simulink model "preliminaryModel_noBS13"  (R2015b)
settings: Solver=FixedStepAuto  StartTime=cmd_time(1215)  StopTime=cmd_time(1215)+10  FixedStep=1E-2  MaxStep=0.08  RelTol=1e-3
values from neighbouring files (symbols this model uses):
  act_0 = 0.3    [runfirst13.m]
  b = 1.365    [runfirst13.m]
  cbar = 0.5    [runfirst13.m]
  CD_alpha = 0.173    [runfirst13.m]
  CD_beta = 0    [runfirst13.m]
  CD_ca = 0    [runfirst13.m]
  CD_el = 0    [runfirst13.m]
  CG = [Xcg Ycg Zcg]    [runfirst13.m]
  CL_alpha = 3.137    [runfirst13.m]
  Cl_alpha = 0    [runfirst13.m]
  Cl_beta = 0.046    [runfirst13.m]
  CL_beta = 0    [runfirst13.m]
  CL_ca = 0.000    (= 0)    [runfirst13.m]
  Cl_ca = 0.000    (= 0)    [runfirst13.m]
  CL_el = 0.000    (= 0)    [runfirst13.m]
  Cl_el = 0.111    [runfirst13.m]
  Cm_alpha = -0.083    [runfirst13.m]
  Cm_beta = 0    [runfirst13.m]
  Cm_ca = -0.456    [runfirst13.m]
  Cm_el = 0.000    (= 0)    [runfirst13.m]
  Cn_alpha = 0    [runfirst13.m]
  Cn_beta = 0    [runfirst13.m]
  Cn_ca = 0.000    (= 0)    [runfirst13.m]
  Cn_el = 0.037    [runfirst13.m]
  CP = [xa_ref 0 0]    [runfirst13.m]
  CY_alpha = 0    [runfirst13.m]
  CY_beta = -0.351    [runfirst13.m]
  CY_ca = 0.000    (= 0)    [runfirst13.m]
  CY_el = 0.049    [runfirst13.m]
  deg_2_rad = 1/rad_2_deg    (= 0.0174532925199)    [runfirst13.m]
  eul_0 = [phi_0 theta_0 psi_0]    [runfirst13.m]
  f = 1/196.877360    (= 0.00507930419221)    [runfirst13.m]
  F_0 = [100 0 0]    [runfirst13.m]
  g = 9.82    [runfirst13.m]
  h_ref = 0    [runfirst13.m]
  heading_0 = 0    [runfirst13.m]
  Iyy = 0.01    [runfirst13.m]
  LL0 = [1 0]    [runfirst13.m]
  m_dot = 0.2    [runfirst13.m]
  mass = W_oew    (= 14.95)    [runfirst13.m]
  mass_e = 0    [runfirst13.m]
  mass_f = mass+W_if    (= 17.85)    [runfirst13.m]
  maxdef_act = 2.0    (= 2)    [runfirst13.m]
  maxrate_act = inf    [runfirst13.m]
  mindef_act = -2.0    (= -2)    [runfirst13.m]
  P_g = 100000    [runfirst13.m]
  pos3_0 = [Xe_0 Ze_0]    [runfirst13.m]
  pos_0 = [Xe_0 Ye_0 Ze_0]    [runfirst13.m]
  q_0 = 0.5    [runfirst13.m]
  R = 287    [runfirst13.m]
  rad_2_deg = 180/pi    (= 57.2957795131)    [runfirst13.m]
  rho_ref = 1.225    [runfirst13.m]
  rot_0 = [p_0 q_0 r_0]    [runfirst13.m]
  S_ref = 0.747    [runfirst13.m]
  T_g = 293    [runfirst13.m]
  theta_0 = 0.02    [runfirst13.m]
  U_0 = 10    [runfirst13.m]
  Vb_0 = [U_0 v_0 w_0]    [runfirst13.m]
  Vw_0 = [uw_0 vw_0 ww_0]    [runfirst13.m]
  w_0 = 0    [runfirst13.m]
  wn_act = 1.7    [runfirst13.m]
  z_act = 0.57    [runfirst13.m]
undefined symbols (not defined in the file or in its folder): Newton, Raphson, U0, w0
libraries: simulink x6
(part 1 of 2)
settings Model: Creator=Victor  LastModifiedBy=victorohman
settings OptimizationCC: BlockReduction=off  UseDivisionForNetSlopeComputation=on  EfficientFloat2IntCast=on
settings DebuggingCC: SignalInfNanChecking=error  SignalRangeChecking=error  ReadBeforeWriteMsg=EnableAllAsError  WriteAfterWriteMsg=EnableAllAsError  WriteAfterReadMsg=EnableAllAsError  AlgebraicLoopMsg=error  ArtificialAlgebraicLoopMsg=error  BlockPriorityViolationMsg=error  SolverPrmCheckMsg=error  InheritedTsInSrcMsg=error  SigSpecEnsureSampleTimeMsg=error  CheckMatrixSingularityMsg=error  IntegerOverflowMsg=error  ParameterUnderflowMsg=error  ParameterPrecisionLossMsg=error  ParameterTunabilityLossMsg=error  UnderSpecifiedDataTypeMsg=error  UnnecessaryDatatypeConvMsg=warning  SignalLabelMismatchMsg=error  UnconnectedInputMsg=error  UnconnectedOutputMsg=error  UnconnectedLineMsg=error  UniqueDataStoreMsg=error  BusObjectLabelMismatch=error  RootOutportRequireBusObject=error  AssertControl=DisableAll  UnknownTsInhSupMsg=error  StateNameClashWarn=warning  StrictBusMsg=ErrorOnBusTreatedAsVector
settings GRTTargetCC: UtilityFuncGeneration=Shared location

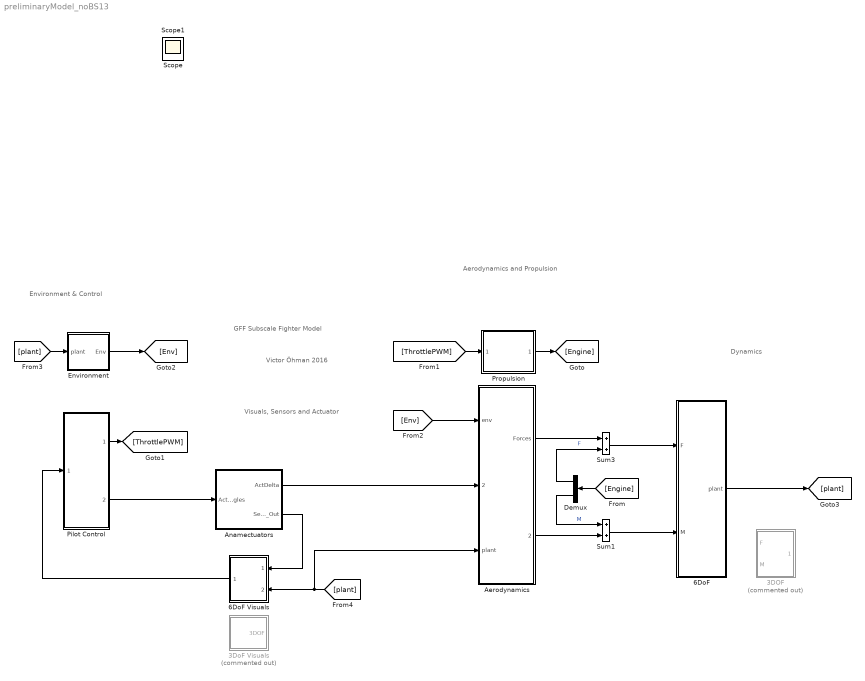
== system preliminaryModel_noBS13 ==
  note: Victor Öhman
      | 2016
  note: GFF
      | Subscale Fighter Model
  note: Environment & Control
  note: Visuals, Sensors
      | and Actuator
  note: Aerodynamics
      | and Propulsion
  note: Dynamics
  3DOF : Subsystem  Commented=on  VariantControl=Variant1
  3DoF Visuals : Subsystem  Commented=on
  6DoF : Subsystem
  6DoF Visuals : Subsystem
  Aerodynamics : Subsystem
  Anamectuators : Subsystem
  Demux : Demux  Outputs=2
  Environment : Subsystem
  Pilot Control : Subsystem
  Propulsion : Subsystem
  Sum1 : Sum  SaturateOnIntegerOverflow=on  InputSameDT=on  OutDataTypeStr=Inherit: Same as first input
  Sum3 : Sum  SaturateOnIntegerOverflow=on  InputSameDT=on  OutDataTypeStr=Inherit: Same as first input
  Scope : Scope
  Scope1 : Scope
  wires:
  Pilot Control/2(ActPos) -> Anamectuators/1(ActCmdAngles)
  Anamectuators/2(Sensor_Out) -> 6DoF Visuals/1(Sensors)
  Propulsion/1(Engine) -> [Engine]
  Aerodynamics/2(Moments) -> Sum1/2
  Aerodynamics/1(Forces) -> Sum3/1
  Demux/1 -> Sum3/2  "F"
  Demux/2 -> Sum1/1  "M"
  Anamectuators/1(ActDelta) -> Aerodynamics/2(ActDelta)
  Sum1/1 -> 6DoF/2(M)
  Sum3/1 -> 6DoF/1(F)
  [Engine] -> Demux/1
  Pilot Control/1(Throttle,PWM) -> [ThrottlePWM]
  [ThrottlePWM] -> Propulsion/1(Throttle)
  Environment/1(Env) -> [Env]
  [Env] -> Aerodynamics/1(env)
  6DoF/1(plant) -> [plant]
  [plant] -> Environment/1(plant)
  [plant] -> Aerodynamics/3(plant), 6DoF Visuals/2(6DOF)
  6DoF Visuals/1(Autopilot) -> Pilot Control/1(Autopilot)

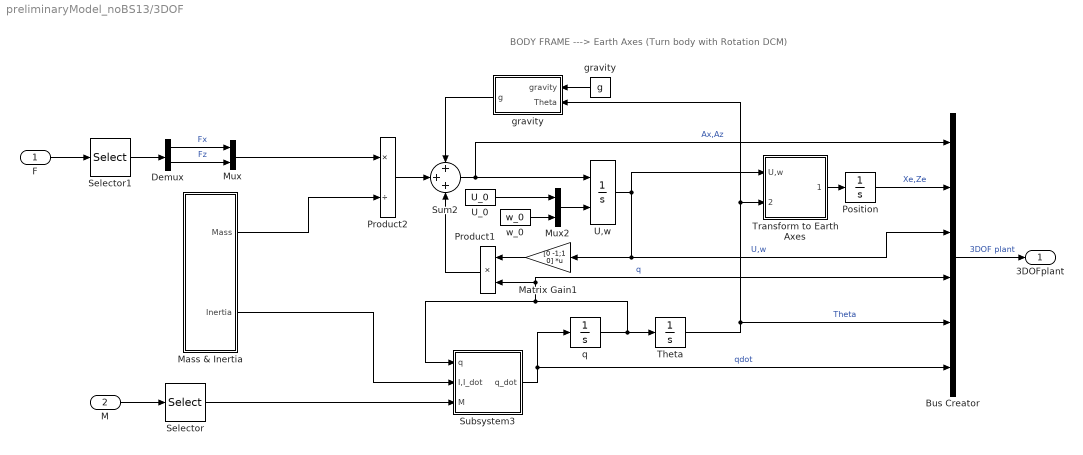
== system preliminaryModel_noBS13/3DOF ==
  note: BODY FRAME ---> Earth Axes (Turn body with Rotation DCM)
  F : Inport
  M : Inport  Port=2
  Bus Creator : BusCreator  Inputs=6
  Demux : Demux  Outputs=2
  Mass & Inertia : Subsystem
  Matrix Gain1 : Gain  Gain=[0 -1;1 0]  Multiplication=Matrix(K*u)  SaturateOnIntegerOverflow=on  OutDataTypeStr=Inherit: Same as input  ParamDataTypeStr=Inherit: Same as input
  Mux : Mux  Inputs=2
  Mux2 : Mux  Inputs=2
  Position : Integrator  InitialCondition=pos3_0
  Product1 : Product  SaturateOnIntegerOverflow=on  InputSameDT=on  OutDataTypeStr=Inherit: Same as first input
  Product2 : Product  Inputs=*/  SaturateOnIntegerOverflow=on  OutDataTypeStr=Inherit: Same as first input
  Selector : Selector  IndexMode=Zero-based  InputPortWidth=3  IndexOptions=Index vector (dialog)  Indices=1  OutputSizes=1
  Selector1 : Selector  InputPortWidth=3  IndexOptions=Index vector (dialog)  Indices=[1 3]  OutputSizes=1
  Subsystem3 : Subsystem
  Sum2 : Sum  Inputs=+++  SaturateOnIntegerOverflow=on
  Theta : Integrator  InitialCondition=theta_0
  Transform to Earth Axes : Subsystem
  U,w : Integrator  InitialConditionSource=external  InitialCondition=convvel([U0 w0],'m/s','m/s')
  U_0 : Constant  Value=U_0
  gravity : Constant  Value=g  OutDataTypeStr=Inherit: Inherit via back propagation
  "gravity " : Subsystem
  q : Integrator  InitialCondition=q_0
  w_0 : Constant  Value=w_0
  3DOFplant : Outport
  wires:
  Bus Creator/1 -> 3DOFplant/1  "3DOF plant"
  Mux2/1 -> U,w/2
  U_0/1 -> Mux2/1
  w_0/1 -> Mux2/2
  Selector/1 -> Subsystem3/3(M)
  U,w/1 -> Matrix Gain1/1, Bus Creator/3, Transform to Earth Axes/1(U,w)  "U,w"
  gravity/1 -> "gravity "/1(gravity)
  Mass & Inertia/2(Inertia) -> Subsystem3/2(I,I_dot)
  Mass & Inertia/1(Mass) -> Product2/2
  Sum2/1 -> U,w/1, Bus Creator/1  "Ax,Az"
  q/1 -> Subsystem3/1(q), Product1/2, Bus Creator/4, Theta/1  "q"
  Subsystem3/1(q_dot) -> q/1, Bus Creator/6  "qdot"
  Theta/1 -> "gravity "/2(Theta), Transform to Earth Axes/2(Theta), Bus Creator/5  "Theta"
  Position/1 -> Bus Creator/2  "Xe,Ze"
  Matrix Gain1/1 -> Product1/1
  Transform to Earth Axes/1(Ue,we) -> Position/1
  Product1/1 -> Sum2/3
  Product2/1 -> Sum2/2
  "gravity "/1(g) -> Sum2/1
  Mux/1 -> Product2/1
  Selector1/1 -> Demux/1
  Demux/2 -> Mux/2  "Fz"
  Demux/1 -> Mux/1  "Fx"
  F/1 -> Selector1/1
  M/1 -> Selector/1

== system preliminaryModel_noBS13/3DoF Visuals ==
  3DOF : Inport
  Bus Selector1 : BusSelector  OutputSignals=Xe;Ze
  Mux1 : Mux  Inputs=1
  To File : ToFile  Filename=output_3dof.mat  SaveFormat=Timeseries
  lat : Scope
  wires:
  3DOF/1 -> Bus Selector1/1
  Mux1/1 -> To File/1
  Bus Selector1/1 -> lat/1, Mux1/1  "<Xe;Ze>"

== system preliminaryModel_noBS13/6DoF ==
  F : Inport
  M : Inport  Port=2
  "  " : Subsystem
  "        " : Subsystem
  "               " : Subsystem
  " 1" : Subsystem
  6DOF : Subsystem
  Bus Creator : BusCreator  Inputs=9
  plant : Outport
  wires:
  F/1 -> 6DOF/1(F)
  "  "/1(body angles) -> Bus Creator/3
  " 1"/1(NED pos) -> Bus Creator/9  "NED pos"
  Bus Creator/1 -> plant/1
  6DOF/8(Xe) -> Bus Creator/8, " 1"/1(Xe)  "Xe"
  "        "/1(omega) -> Bus Creator/5  "w"
  6DOF/1(Ve) -> Bus Creator/1  "Ve"
  6DOF/7(Ab) -> Bus Creator/7  "Ab"
  "               "/1(omegadot) -> Bus Creator/6  "wdot"
  6DOF/2(Vb) -> Bus Creator/2  "Vb"
  6DOF/3(Euler) -> "  "/1(phi,theta,psi)
  6DOF/6(pdot,qdot,rdot) -> "               "/1(pdot,qdot,rdot)
  6DOF/4(DCM) -> Bus Creator/4  "DCM"
  6DOF/5(p,q,r) -> "        "/1(p,q,r)
  M/1 -> 6DOF/2(M)

== system preliminaryModel_noBS13/6DoF Visuals ==
  note: Block för att kolla, skicka vidare
  Sensors : Inport
  6DOF : Inport  Port=2
  Bus Selector2 : BusSelector  OutputSignals=NED pos.lat,NED pos.long,NED pos.alt,body angles.phi,body angles.theta,body angles.psi
  Mux1 : Mux  Inputs=3
  Mux2 : Mux  Inputs=3
  Scope : Scope  NumInputPorts=3
  To File : ToFile  Filename=out_pos.mat  MatrixName=out_pos  SaveFormat=Timeseries
  To File1 : ToFile  Filename=out_eul.mat  MatrixName=out_eul  SaveFormat=Timeseries
  alt : Scope
  lat : Scope
  long : Scope
  Autopilot : Outport
  wires:
  Bus Selector2/4 -> Mux2/1, Scope/1  "<phi>"
  Bus Selector2/6 -> Mux2/3, Scope/3  "<psi>"
  6DOF/1 -> Bus Selector2/1
  Bus Selector2/5 -> Mux2/2, Scope/2  "<theta>"
  Bus Selector2/2 -> Mux1/2, long/1  "<long>"
  Bus Selector2/1 -> Mux1/1, lat/1  "<lat>"
  Bus Selector2/3 -> Mux1/3, alt/1  "<alt>"
  Mux1/1 -> To File/1
  Mux2/1 -> To File1/1
  Sensors/1 -> Autopilot/1

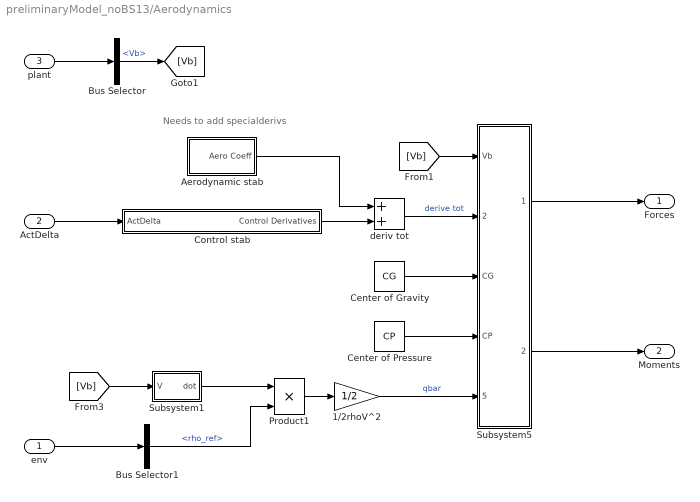
== system preliminaryModel_noBS13/Aerodynamics ==
  note: Needs to add specialderivs
  env : Inport
  ActDelta : Inport  Port=2
  plant : Inport  Port=3
  1/2rhoV^2 : Gain  Gain=1/2  SaturateOnIntegerOverflow=on  OutDataTypeStr=Inherit: Same as input  ParamDataTypeStr=Inherit: Same as input
  Aerodynamic stab : Subsystem
  Bus Selector : BusSelector  OutputSignals=Vb
  Bus Selector1 : BusSelector  OutputSignals=rho_ref
  Center of Gravity : Constant  Value=CG
  Center of Pressure : Constant  Value=CP
  Control stab : Subsystem
  Product1 : Product  SaturateOnIntegerOverflow=on  InputSameDT=on  OutDataTypeStr=Inherit: Same as first input
  Subsystem1 : Subsystem
  Subsystem5 : Subsystem
  deriv tot : Sum  SaturateOnIntegerOverflow=on  InputSameDT=on  OutDataTypeStr=Inherit: Same as first input
  Forces : Outport
  Moments : Outport  Port=2
  wires:
  plant/1 -> Bus Selector/1
  ActDelta/1 -> Control stab/1(ActDelta)
  env/1 -> Bus Selector1/1
  Bus Selector/1 -> [Vb]  "<Vb>"
  Aerodynamic stab/1(Aero Coeff) -> deriv tot/1
  Control stab/1(Control Derivatives) -> deriv tot/2
  Bus Selector1/1 -> Product1/2  "<rho_ref>"
  Product1/1 -> 1/2rhoV^2/1
  Subsystem1/1(dot) -> Product1/1
  [Vb] -> Subsystem1/1(V)
  Center of Gravity/1 -> Subsystem5/3(CG)
  deriv tot/1 -> Subsystem5/2(coef)  "derive tot"
  Center of Pressure/1 -> Subsystem5/4(CP)
  1/2rhoV^2/1 -> Subsystem5/5(qbar)  "qbar"
  Subsystem5/2(Moments) -> Moments/1
  Subsystem5/1(Forces) -> Forces/1
  [Vb] -> Subsystem5/1(Vb)

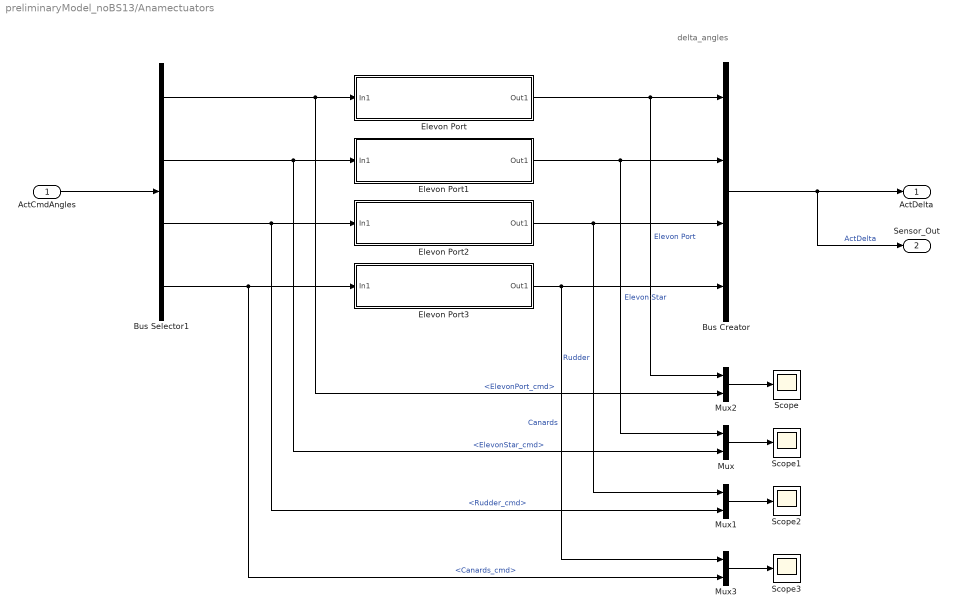
== system preliminaryModel_noBS13/Anamectuators ==
  note: delta_angles
  ActCmdAngles : Inport
  Bus Creator : BusCreator  Inputs=4
  Bus Selector1 : BusSelector  OutputSignals=ElevonPort_cmd,ElevonStar_cmd,Rudder_cmd,Canards_cmd
  Elevon Port : Subsystem
  Elevon Port1 : Subsystem
  Elevon Port2 : Subsystem
  Elevon Port3 : Subsystem
  Mux{,1..3} (4 alike) : Mux  Inputs=2
  Scope{,1..3} (4 alike) : Scope
  ActDelta : Outport
  Sensor_Out : Outport  Port=2
  wires:
  ActCmdAngles/1 -> Bus Selector1/1
  Bus Selector1/1 -> Elevon Port/1(In1), Mux2/2  "<ElevonPort_cmd>"
  Bus Selector1/2 -> Elevon Port1/1(In1), Mux/2  "<ElevonStar_cmd>"
  Bus Selector1/3 -> Elevon Port2/1(In1), Mux1/2  "<Rudder_cmd>"
  Bus Creator/1 -> Sensor_Out/1, ActDelta/1  "ActDelta"
  Mux/1 -> Scope1/1
  Mux1/1 -> Scope2/1
  Mux2/1 -> Scope/1
  Mux3/1 -> Scope3/1
  Bus Selector1/4 -> Elevon Port3/1(In1), Mux3/2  "<Canards_cmd>"
  Elevon Port/1(Out1) -> Bus Creator/1, Mux2/1  "Elevon Port"
  Elevon Port1/1(Out1) -> Bus Creator/2, Mux/1  "Elevon Star"
  Elevon Port2/1(Out1) -> Bus Creator/3, Mux1/1  "Rudder"
  Elevon Port3/1(Out1) -> Bus Creator/4, Mux3/1  "Canards"

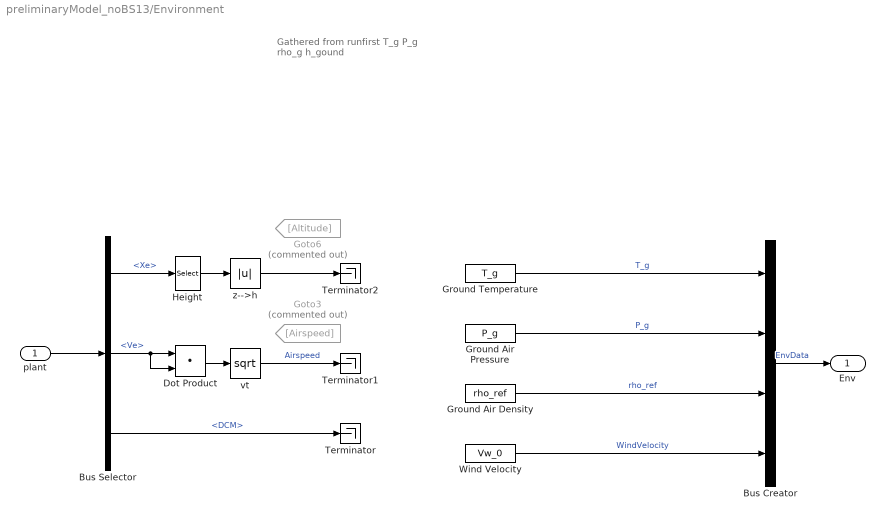
== system preliminaryModel_noBS13/Environment ==
  note: Gathered from runfirst
      | T_g
      | P_g
      | rho_g
      | h_gound
  plant : Inport
  Bus Creator : BusCreator  Inputs='T_g','P_g','rho_ref','WindVelocity'
  Bus Selector : BusSelector  OutputSignals=Xe,Ve,DCM
  Dot Product : DotProduct  OutDataTypeStr=Inherit: Inherit via internal rule
  Goto3 : Goto  Commented=on  GotoTag=Airspeed
  Goto6 : Goto  Commented=on  GotoTag=Altitude
  Ground Air Density : Constant  Value=rho_ref
  Ground Air Pressure : Constant  Value=P_g
  Ground Temperature : Constant  Value=T_g
  Height : Selector  InputPortWidth=3  IndexOptions=Index vector (dialog)  Indices=[3]  OutputSizes=1
  Terminator : Terminator
  Terminator1 : Terminator
  Terminator2 : Terminator
  Wind Velocity : Constant  Value=Vw_0
  vt : Math  Operator=sqrt  SaturateOnIntegerOverflow=on
  z-->h : Abs  SaturateOnIntegerOverflow=on
  Env : Outport  InitialOutput=0
  wires:
  Bus Creator/1 -> Env/1  "EnvData"
  Ground Temperature/1 -> Bus Creator/1  "T_g"
  Ground Air Pressure/1 -> Bus Creator/2  "P_g"
  Bus Selector/3 -> Terminator/1  "<DCM>"
  Height/1 -> z-->h/1
  Ground Air Density/1 -> Bus Creator/3  "rho_ref"
  z-->h/1 -> Terminator2/1
  Bus Selector/1 -> Height/1  "<Xe>"
  plant/1 -> Bus Selector/1
  vt/1 -> Terminator1/1  "Airspeed"
  Dot Product/1 -> vt/1
  Wind Velocity/1 -> Bus Creator/4  "WindVelocity"
  Bus Selector/2 -> Dot Product/2, Dot Product/1  "<Ve>"

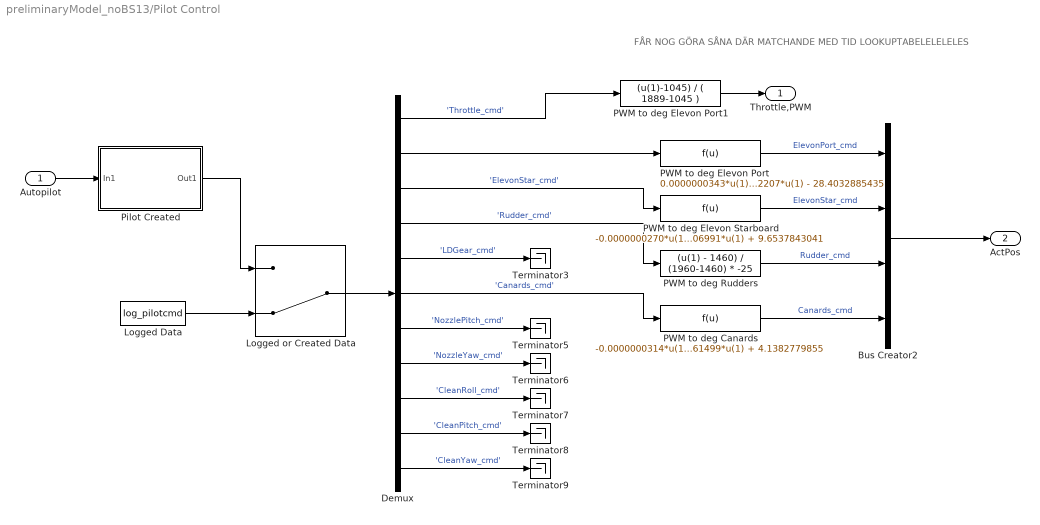
== system preliminaryModel_noBS13/Pilot Control ==
  note: FÅR NOG GÖRA SÅNA DÄR MATCHANDE MED TID LOOKUPTABELELELELES
  Autopilot : Inport
  Bus Creator2 : BusCreator  Inputs=4
  Demux : Demux  Outputs=11
  Logged Data : FromWorkspace  VariableName=log_pilotcmd  SampleTime=0
  Logged or Created Data : ManualSwitch  CurrentSetting=0
  PWM to deg Canards : Fcn  Expr=-0.0000000314*u(1)^3 + 0.0001339606*u(1)^2 - 0.1313561499*u(1) + 4.1382779855
  PWM to deg Elevon Port : Fcn  Expr=0.0000000343*u(1)^3 - 0.0001530183*u(1)^2 + 0.1711412207*u(1) - 28.4032885435
  PWM to deg Elevon Port1 : Fcn  Expr=(u(1)-1045) / ( 1889-1045 )
  PWM to deg Elevon Starboard : Fcn  Expr=-0.0000000270*u(1)^3 + 0.0001190841*u(1)^2 - 0.1226606991*u(1) + 9.6537843041
  PWM to deg Rudders : Fcn  Expr=(u(1) - 1460) / (1960-1460) * -25
  Pilot Created : Subsystem
  Terminator{3,5..9} (6 alike) : Terminator
  Throttle,PWM : Outport
  ActPos : Outport  Port=2
  wires:
  Bus Creator2/1 -> ActPos/1
  PWM to deg Canards/1 -> Bus Creator2/4  "Canards_cmd"
  PWM to deg Elevon Port/1 -> Bus Creator2/1  "ElevonPort_cmd"
  PWM to deg Elevon Starboard/1 -> Bus Creator2/2  "ElevonStar_cmd"
  PWM to deg Rudders/1 -> Bus Creator2/3  "Rudder_cmd"
  Logged Data/1 -> Logged or Created Data/2
  Demux/1 -> PWM to deg Elevon Port1/1  "'Throttle_cmd'"
  Demux/2 -> PWM to deg Elevon Port/1
  Demux/3 -> PWM to deg Elevon Starboard/1  "'ElevonStar_cmd'"
  Demux/4 -> PWM to deg Rudders/1  "'Rudder_cmd'"
  Demux/5 -> Terminator3/1  "'LDGear_cmd'"
  Demux/6 -> PWM to deg Canards/1  "'Canards_cmd'"
  Demux/7 -> Terminator5/1  "'NozzlePitch_cmd'"
  Demux/8 -> Terminator6/1  "'NozzleYaw_cmd'"
  Demux/9 -> Terminator7/1  "'CleanRoll_cmd'"
  Demux/10 -> Terminator8/1  "'CleanPitch_cmd'"
  Demux/11 -> Terminator9/1  "'CleanYaw_cmd'"
  Logged or Created Data/1 -> Demux/1
  Pilot Created/1(Out1) -> Logged or Created Data/1
  Autopilot/1 -> Pilot Created/1(In1)
  PWM to deg Elevon Port1/1 -> Throttle,PWM/1

== system preliminaryModel_noBS13/Propulsion ==
  Throttle : Inport
  Engine Input : Subsystem
      settings: RTWSystemCode=Inline
  Mux4 : Mux  Inputs=2
  Engine : Outport
  wires:
  Throttle/1 -> Engine Input/1(throttle)
  Engine Input/2(M) -> Mux4/2
  Engine Input/1(F) -> Mux4/1
  Mux4/1 -> Engine/1

== system preliminaryModel_noBS13/3DOF/Mass & Inertia ==
  Constant : Constant  Value=Iyy  OutDataTypeStr=double
  Constant2 : Constant  Value=0  OutDataTypeStr=double
  Mux1 : Mux  Inputs=2
  mass1 : Integrator  InitialCondition=mass  LimitOutput=on  UpperSaturationLimit=mass_f  LowerSaturationLimit=mass_e
  massflow : Constant  Value=m_dot  OutDataTypeStr=Inherit: Inherit via back propagation
  Mass : Outport
  Inertia : Outport  Port=2
  wires:
  Constant2/1 -> Mux1/2
  Constant/1 -> Mux1/1
  massflow/1 -> mass1/1
  Mux1/1 -> Inertia/1
  mass1/1 -> Mass/1

== system preliminaryModel_noBS13/3DOF/Subsystem3 ==
  q : Inport
  I,I_dot : Inport  Port=2
  M : Inport  Port=3
  Demux : Demux  Outputs=2
  Product3 : Product  Inputs=*/  SaturateOnIntegerOverflow=on  InputSameDT=on  OutDataTypeStr=Inherit: Same as first input
  Product4 : Product  SaturateOnIntegerOverflow=on  InputSameDT=on  OutDataTypeStr=Inherit: Same as first input
  Sum2 : Sum  Inputs=|+-  SaturateOnIntegerOverflow=on
  q_dot : Outport
  wires:
  Demux/2 -> Product4/1
  I,I_dot/1 -> Demux/1
  Product4/1 -> Sum2/2
  q/1 -> Product4/2
  M/1 -> Sum2/1
  Product3/1 -> q_dot/1
  Demux/1 -> Product3/2
  Sum2/1 -> Product3/1

== system preliminaryModel_noBS13/3DOF/Transform to Earth Axes ==
  note: Rotation order ZYX
  U,w : Inport
  Theta : Inport  Port=2
  Constant : Constant  Value=0
  Mux3 : Mux  Inputs=3
  Mux4 : Mux  Inputs=3
  Product : Product  Multiplication=Matrix(*)  SaturateOnIntegerOverflow=on  OutDataTypeStr=Inherit: Same as first input
  Rotation Angles to Direction Cosine Matrix : Subsystem
  Selector : Selector  IndexMode=Zero-based  InputPortWidth=2  IndexOptions=Index vector (dialog)  Indices=0  OutputSizes=1
  Selector1 : Selector  InputPortWidth=3  IndexOptions=Index vector (dialog)  Indices=[1 3]  OutputSizes=1
  Selector2 : Selector  InputPortWidth=2  IndexOptions=Index vector (dialog)  Indices=2  OutputSizes=1
  Transpose : Math  Operator=transpose  SaturateOnIntegerOverflow=on
  Ue,we : Outport
  wires:
  Selector/1 -> Mux4/1
  Mux4/1 -> Product/2
  Transpose/1 -> Product/1  "DCMeb"
  Product/1 -> Selector1/1
  Theta/1 -> Mux3/2
  Rotation Angles to Direction Cosine Matrix/1(DCMbe) -> Transpose/1
  Mux3/1 -> Rotation Angles to Direction Cosine Matrix/1("[R1,R2,R3]")
  Selector1/1 -> Ue,we/1
  U,w/1 -> Selector/1, Selector2/1
  Selector2/1 -> Mux4/3
  Constant/1 -> Mux3/1, Mux3/3, Mux4/2

== system preliminaryModel_noBS13/3DOF/gravity  ==
  gravity : Inport
  Theta : Inport  Port=2
  Mux : Mux  Inputs=2
  Product : Product  SaturateOnIntegerOverflow=on  InputSameDT=on  OutDataTypeStr=Inherit: Same as first input
  Unary Minus : UnaryMinus
  sincos : Trigonometry  Operator=sincos
  g : Outport
  wires:
  sincos/1 -> Unary Minus/1
  sincos/2 -> Mux/2
  gravity/1 -> Product/2
  Theta/1 -> sincos/1
  Mux/1 -> Product/1
  Product/1 -> g/1
  Unary Minus/1 -> Mux/1

== system preliminaryModel_noBS13/6DoF/   ==
  phi,theta,psi : Inport
  Bus Creator1 : BusCreator  Inputs=3
  Demux3 : Demux  Outputs=3
  body angles : Outport
  wires:
  Demux3/2 -> Bus Creator1/2  "theta"
  Bus Creator1/1 -> body angles/1  "body angles"
  Demux3/3 -> Bus Creator1/3  "psi"
  phi,theta,psi/1 -> Demux3/1
  Demux3/1 -> Bus Creator1/1  "phi"

== system preliminaryModel_noBS13/6DoF/         ==
  p,q,r : Inport
  Bus Creator2 : BusCreator  Inputs=3
  Demux1 : Demux  Outputs=3
  omega : Outport
  wires:
  p,q,r/1 -> Demux1/1
  Bus Creator2/1 -> omega/1
  Demux1/3 -> Bus Creator2/3  "r"
  Demux1/1 -> Bus Creator2/1  "p"
  Demux1/2 -> Bus Creator2/2  "q"

== system preliminaryModel_noBS13/6DoF/                ==
  pdot,qdot,rdot : Inport
  Bus Creator2 : BusCreator  Inputs=3
  Demux1 : Demux  Outputs=3
  omegadot : Outport
  wires:
  pdot,qdot,rdot/1 -> Demux1/1
  Bus Creator2/1 -> omegadot/1
  Demux1/3 -> Bus Creator2/3  "rdot"
  Demux1/1 -> Bus Creator2/1  "pdot"
  Demux1/2 -> Bus Creator2/2  "qdot"

== system preliminaryModel_noBS13/6DoF/ 1 ==
  Xe : Inport
  Bus Creator : BusCreator  Inputs=3
  Constant : Constant  Value=h_ref
  Demux2 : Demux  Outputs=2
  Flat Earth to LLA : Subsystem
  NED pos : Outport
  wires:
  Xe/1 -> Flat Earth to LLA/1(Xe)
  Bus Creator/1 -> NED pos/1
  Constant/1 -> Flat Earth to LLA/2(ground height)
  Flat Earth to LLA/2(h) -> Bus Creator/3  "alt"
  Flat Earth to LLA/1(mu l) -> Demux2/1
  Demux2/1 -> Bus Creator/1  "lat"
  Demux2/2 -> Bus Creator/2  "long"

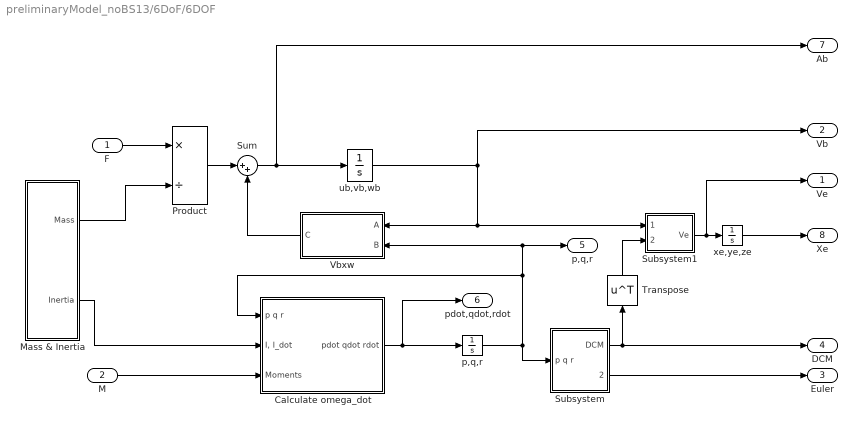
== system preliminaryModel_noBS13/6DoF/6DOF ==
  F : Inport
  M : Inport  Port=2
  Calculate omega_dot : Subsystem
  Mass & Inertia : Subsystem
  Product : Product  Inputs=*/  SaturateOnIntegerOverflow=on  OutDataTypeStr=Inherit: Same as first input
  Subsystem : Subsystem
  Subsystem1 : Subsystem
  Sum : Sum  Inputs=|++  SaturateOnIntegerOverflow=on
  Transpose : Math  Operator=transpose  SaturateOnIntegerOverflow=on
  Vbxw : Subsystem
  "p,q,r " : Integrator  InitialCondition=rot_0
  ub,vb,wb : Integrator  InitialCondition=Vb_0
  xe,ye,ze : Integrator  InitialCondition=pos_0
  Ve : Outport
  Vb : Outport  Port=2
  Euler : Outport  Port=3
  DCM : Outport  Port=4
  p,q,r : Outport  Port=5
  pdot,qdot,rdot : Outport  Port=6
  Ab : Outport  Port=7
  Xe : Outport  Port=8
  wires:
  Subsystem1/1(Ve) -> Ve/1, xe,ye,ze/1
  Sum/1 -> Ab/1, ub,vb,wb/1
  ub,vb,wb/1 -> Vb/1, Subsystem1/1(x y z), Vbxw/1(A)
  Calculate omega_dot/1(pdot qdot rdot) -> pdot,qdot,rdot/1, "p,q,r "/1
  Transpose/1 -> Subsystem1/2(transform coefficients)
  Subsystem/1(DCM) -> Transpose/1, DCM/1
  Product/1 -> Sum/1
  M/1 -> Calculate omega_dot/3(Moments)
  "p,q,r "/1 -> Subsystem/1("p q r "), p,q,r/1, Vbxw/2(B), Calculate omega_dot/1(p q r)
  xe,ye,ze/1 -> Xe/1
  Vbxw/1(C) -> Sum/2
  Subsystem/2(Euler) -> Euler/1
  Mass & Inertia/1(Mass) -> Product/2
  F/1 -> Product/1
  Mass & Inertia/2(Inertia) -> Calculate omega_dot/2("I, I_dot")

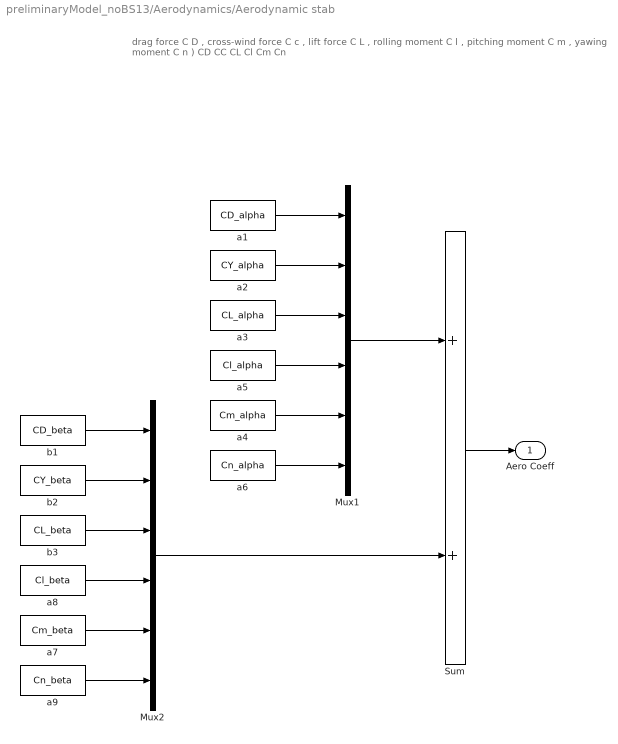
== system preliminaryModel_noBS13/Aerodynamics/Aerodynamic stab ==
  note: drag force C D , cross-wind force C c , lift force C L , rolling moment C l , pitching moment C m , yawing moment C n )
      | CD
      | CC
      | CL
      | Cl
      | Cm
      | Cn
  Mux1 : Mux  Inputs=6
  Mux2 : Mux  Inputs=6
  Sum : Sum  Inputs=2  SaturateOnIntegerOverflow=on  InputSameDT=on  OutDataTypeStr=Inherit: Same as first input
  a1 : Constant  Value=CD_alpha
  a2 : Constant  Value=CY_alpha
  a3 : Constant  Value=CL_alpha
  a4 : Constant  Value=Cm_alpha
  a5 : Constant  Value=Cl_alpha
  a6 : Constant  Value=Cn_alpha
  a7 : Constant  Value=Cm_beta
  a8 : Constant  Value=Cl_beta
  a9 : Constant  Value=Cn_beta
  b1 : Constant  Value=CD_beta
  b2 : Constant  Value=CY_beta
  b3 : Constant  Value=CL_beta
  Aero Coeff : Outport  InitialOutput=0
  wires:
  a1/1 -> Mux1/1
  a2/1 -> Mux1/2
  a4/1 -> Mux1/5
  a3/1 -> Mux1/3
  b1/1 -> Mux2/1
  b2/1 -> Mux2/2
  b3/1 -> Mux2/3
  Sum/1 -> Aero Coeff/1
  Mux1/1 -> Sum/1
  Mux2/1 -> Sum/2
  a5/1 -> Mux1/4
  a6/1 -> Mux1/6
  a8/1 -> Mux2/4
  a7/1 -> Mux2/5
  a9/1 -> Mux2/6

== system preliminaryModel_noBS13/Aerodynamics/Control stab ==
  note: delta angles in
  ActDelta : Inport
  Bus Selector : BusSelector  OutputSignals=Canards,Elevon Port,Elevon Star,Rudder
  Subsystem : Subsystem
  Control Derivatives : Outport
  wires:
  ActDelta/1 -> Bus Selector/1
  Bus Selector/2 -> Subsystem/2(Elevon 1)  "<Elevon Port>"
  Subsystem/1(Control Derivatives) -> Control Derivatives/1
  Bus Selector/3 -> Subsystem/3(Elevon 2)  "<Elevon Star>"
  Bus Selector/4 -> Subsystem/4(Rudder)  "<Rudder>"
  Bus Selector/1 -> Subsystem/1(Canard Actions)  "<Canards>"

== system preliminaryModel_noBS13/Aerodynamics/Subsystem1 ==
  V : Inport
  Demux2 : Demux  Outputs=3
  Product : Product  RndMeth=Zero
  Product5 : Product  RndMeth=Zero
  Product6 : Product  RndMeth=Zero
  Sum2 : Sum  Inputs=+++
  dot : Outport
  wires:
  Demux2/3 -> Product6/2, Product6/1
  Demux2/2 -> Product5/1, Product5/2
  Sum2/1 -> dot/1
  Product6/1 -> Sum2/3
  Product/1 -> Sum2/1
  Demux2/1 -> Product/2, Product/1
  V/1 -> Demux2/1
  Product5/1 -> Sum2/2

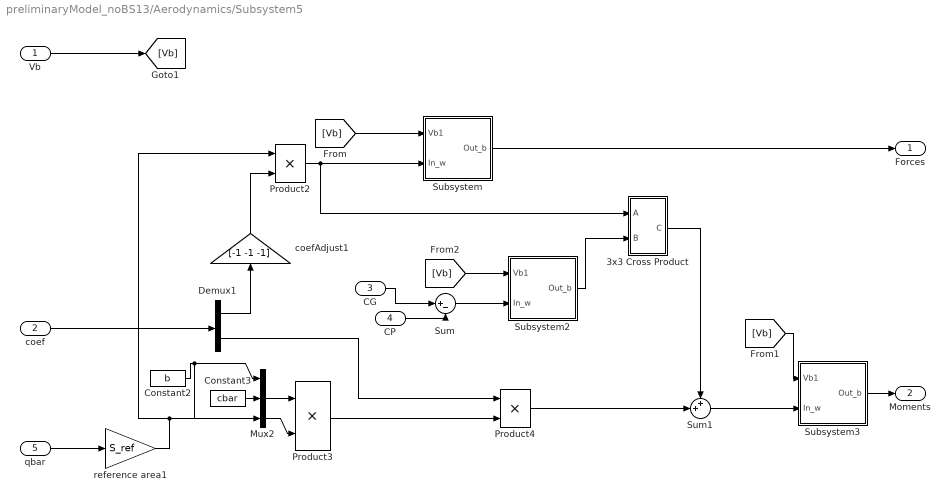
== system preliminaryModel_noBS13/Aerodynamics/Subsystem5 ==
  Vb : Inport
  coef : Inport  Port=2
  CG : Inport  Port=3
  CP : Inport  Port=4
  qbar : Inport  Port=5
  3x3 Cross Product : Subsystem
  Constant2 : Constant  Value=b
  Constant3 : Constant  Value=cbar
  Demux1 : Demux  Outputs=[3,3]
  Mux2 : Mux  Inputs=3
  Product2 : Product  SaturateOnIntegerOverflow=on  InputSameDT=on  OutDataTypeStr=Inherit: Same as first input
  Product3 : Product  SaturateOnIntegerOverflow=on  InputSameDT=on  OutDataTypeStr=Inherit: Same as first input
  Product4 : Product  SaturateOnIntegerOverflow=on  InputSameDT=on  OutDataTypeStr=Inherit: Same as first input
  Subsystem : Subsystem
  Subsystem2 : Subsystem
  Subsystem3 : Subsystem
  Sum : Sum  Inputs=|+-  SaturateOnIntegerOverflow=on
  Sum1 : Sum  Inputs=++|  SaturateOnIntegerOverflow=on  InputSameDT=on  OutDataTypeStr=Inherit: Same as first input
  coefAdjust1 : Gain  Gain=[-1 -1 -1]
  reference area1 : Gain  Gain=S_ref  SaturateOnIntegerOverflow=on  OutDataTypeStr=Inherit: Same as input  ParamDataTypeStr=Inherit: Same as input
  Forces : Outport
  Moments : Outport  Port=2
  wires:
  coef/1 -> Demux1/1
  qbar/1 -> reference area1/1
  Sum/1 -> Subsystem2/2(In_w)
  Mux2/1 -> Product3/1
  Product3/1 -> Product4/2
  Demux1/1 -> coefAdjust1/1
  Product2/1 -> 3x3 Cross Product/1(A), Subsystem/2(In_w)
  Subsystem2/1(Out_b) -> 3x3 Cross Product/2(B)
  [Vb] -> Subsystem2/1(Vb1)
  Constant3/1 -> Mux2/2
  Constant2/1 -> Mux2/1, Mux2/3
  Subsystem3/1(Out_b) -> Moments/1
  CP/1 -> Sum/2
  Demux1/2 -> Product4/1
  3x3 Cross Product/1(C) -> Sum1/1
  coefAdjust1/1 -> Product2/2
  Product4/1 -> Sum1/2
  CG/1 -> Sum/1
  Sum1/1 -> Subsystem3/2(In_w)
  Subsystem/1(Out_b) -> Forces/1
  [Vb] -> Subsystem3/1(Vb1)
  [Vb] -> Subsystem/1(Vb1)
  reference area1/1 -> Product2/1, Product3/2
  Vb/1 -> [Vb]

== system preliminaryModel_noBS13/Anamectuators/Elevon Port ==
  note: 2nd Order Non-linear Actuator
  In1 : Inport
  2*zeta * wn : Gain  Gain=2.0 * z_act* wn_act  SaturateOnIntegerOverflow=on  OutDataTypeStr=Inherit: Same as input  ParamDataTypeStr=Inherit: Same as input
  Demand limits : Saturate  UpperLimit=maxdef_act  LowerLimit=mindef_act
  Limited Deflection : Integrator  InitialCondition=act_0  LimitOutput=on  UpperSaturationLimit=maxdef_act  LowerSaturationLimit=mindef_act
  Servo rate : Integrator
  Sum2 : Sum  Inputs=|+-  SaturateOnIntegerOverflow=on  InputSameDT=on  OutDataTypeStr=Inherit: Same as first input
  Sum3 : Sum  Inputs=|+-  SaturateOnIntegerOverflow=on  InputSameDT=on  OutDataTypeStr=Inherit: Same as first input
  rate limit*2*zeta/wn : Saturate  UpperLimit=maxrate_act*2*z_act/wn_act  LowerLimit=-maxrate_act*2*z_act/wn_act
  wn^2 : Gain  Gain=wn_act* wn_act  SaturateOnIntegerOverflow=on  OutDataTypeStr=Inherit: Same as input  ParamDataTypeStr=Inherit: Same as input
  Out1 : Outport
  wires:
  In1/1 -> Demand limits/1
  wn^2/1 -> Sum2/1
  Sum2/1 -> Servo rate/1
  Servo rate/1 -> 2*zeta * wn/1, Limited Deflection/1
  Sum3/1 -> rate limit*2*zeta/wn/1
  Limited Deflection/1 -> Out1/1, Sum3/2
  Demand limits/1 -> Sum3/1
  rate limit*2*zeta/wn/1 -> wn^2/1
  2*zeta * wn/1 -> Sum2/2

== system preliminaryModel_noBS13/Anamectuators/Elevon Port1 ==
  note: 2nd Order Non-linear Actuator
  In1 : Inport
  2*zeta * wn : Gain  Gain=2.0 * z_act* wn_act  SaturateOnIntegerOverflow=on  OutDataTypeStr=Inherit: Same as input  ParamDataTypeStr=Inherit: Same as input
  Demand limits : Saturate  UpperLimit=maxdef_act  LowerLimit=mindef_act
  Limited Deflection : Integrator  InitialCondition=act_0  LimitOutput=on  UpperSaturationLimit=maxdef_act  LowerSaturationLimit=mindef_act
  Servo rate : Integrator
  Sum2 : Sum  Inputs=|+-  SaturateOnIntegerOverflow=on  InputSameDT=on  OutDataTypeStr=Inherit: Same as first input
  Sum3 : Sum  Inputs=|+-  SaturateOnIntegerOverflow=on  InputSameDT=on  OutDataTypeStr=Inherit: Same as first input
  rate limit*2*zeta/wn : Saturate  UpperLimit=maxrate_act*2*z_act/wn_act  LowerLimit=-maxrate_act*2*z_act/wn_act
  wn^2 : Gain  Gain=wn_act* wn_act  SaturateOnIntegerOverflow=on  OutDataTypeStr=Inherit: Same as input  ParamDataTypeStr=Inherit: Same as input
  Out1 : Outport
  wires:
  In1/1 -> Demand limits/1
  wn^2/1 -> Sum2/1
  Sum2/1 -> Servo rate/1
  Servo rate/1 -> 2*zeta * wn/1, Limited Deflection/1
  Sum3/1 -> rate limit*2*zeta/wn/1
  Limited Deflection/1 -> Out1/1, Sum3/2
  Demand limits/1 -> Sum3/1
  rate limit*2*zeta/wn/1 -> wn^2/1
  2*zeta * wn/1 -> Sum2/2

== system preliminaryModel_noBS13/Anamectuators/Elevon Port2 ==
  note: 2nd Order Non-linear Actuator
  In1 : Inport
  2*zeta * wn : Gain  Gain=2.0 * z_act* wn_act  SaturateOnIntegerOverflow=on  OutDataTypeStr=Inherit: Same as input  ParamDataTypeStr=Inherit: Same as input
  Demand limits : Saturate  UpperLimit=maxdef_act  LowerLimit=mindef_act
  Limited Deflection : Integrator  InitialCondition=act_0  LimitOutput=on  UpperSaturationLimit=maxdef_act  LowerSaturationLimit=mindef_act
  Servo rate : Integrator
  Sum2 : Sum  Inputs=|+-  SaturateOnIntegerOverflow=on  InputSameDT=on  OutDataTypeStr=Inherit: Same as first input
  Sum3 : Sum  Inputs=|+-  SaturateOnIntegerOverflow=on  InputSameDT=on  OutDataTypeStr=Inherit: Same as first input
  rate limit*2*zeta/wn : Saturate  UpperLimit=maxrate_act*2*z_act/wn_act  LowerLimit=-maxrate_act*2*z_act/wn_act
  wn^2 : Gain  Gain=wn_act* wn_act  SaturateOnIntegerOverflow=on  OutDataTypeStr=Inherit: Same as input  ParamDataTypeStr=Inherit: Same as input
  Out1 : Outport
  wires:
  In1/1 -> Demand limits/1
  wn^2/1 -> Sum2/1
  Sum2/1 -> Servo rate/1
  Servo rate/1 -> 2*zeta * wn/1, Limited Deflection/1
  Sum3/1 -> rate limit*2*zeta/wn/1
  Limited Deflection/1 -> Out1/1, Sum3/2
  Demand limits/1 -> Sum3/1
  rate limit*2*zeta/wn/1 -> wn^2/1
  2*zeta * wn/1 -> Sum2/2

== system preliminaryModel_noBS13/Anamectuators/Elevon Port3 ==
  note: 2nd Order Non-linear Actuator
  In1 : Inport
  2*zeta * wn : Gain  Gain=2.0 * z_act* wn_act  SaturateOnIntegerOverflow=on  OutDataTypeStr=Inherit: Same as input  ParamDataTypeStr=Inherit: Same as input
  Demand limits : Saturate  UpperLimit=maxdef_act  LowerLimit=mindef_act
  Limited Deflection : Integrator  InitialCondition=act_0  LimitOutput=on  UpperSaturationLimit=maxdef_act  LowerSaturationLimit=mindef_act
  Servo rate : Integrator
  Sum2 : Sum  Inputs=|+-  SaturateOnIntegerOverflow=on  InputSameDT=on  OutDataTypeStr=Inherit: Same as first input
  Sum3 : Sum  Inputs=|+-  SaturateOnIntegerOverflow=on  InputSameDT=on  OutDataTypeStr=Inherit: Same as first input
  rate limit*2*zeta/wn : Saturate  UpperLimit=maxrate_act*2*z_act/wn_act  LowerLimit=-maxrate_act*2*z_act/wn_act
  wn^2 : Gain  Gain=wn_act* wn_act  SaturateOnIntegerOverflow=on  OutDataTypeStr=Inherit: Same as input  ParamDataTypeStr=Inherit: Same as input
  Out1 : Outport
  wires:
  In1/1 -> Demand limits/1
  wn^2/1 -> Sum2/1
  Sum2/1 -> Servo rate/1
  Servo rate/1 -> 2*zeta * wn/1, Limited Deflection/1
  Sum3/1 -> rate limit*2*zeta/wn/1
  Limited Deflection/1 -> Out1/1, Sum3/2
  Demand limits/1 -> Sum3/1
  rate limit*2*zeta/wn/1 -> wn^2/1
  2*zeta * wn/1 -> Sum2/2

== system preliminaryModel_noBS13/Pilot Control/Pilot Created ==
  In1 : Inport
  Constant : Constant  Value=[1 1 1 1 1 1 1 1 1 1 1]  OutDataTypeStr=double
  Terminator : Terminator
  Out1 : Outport
  wires:
  In1/1 -> Terminator/1
  Constant/1 -> Out1/1

== system preliminaryModel_noBS13/Propulsion/Engine Input ==
  throttle : Inport
  Constant : Constant  Value=F_0
  Constant1 : Constant  Value=[1 1 1]
  Terminator : Terminator
  F : Outport
  M : Outport  Port=2
  wires:
  Constant/1 -> F/1
  Constant1/1 -> M/1
  throttle/1 -> Terminator/1

== system preliminaryModel_noBS13/3DOF/Transform to Earth Axes/Rotation Angles to Direction Cosine Matrix ==
  "[R1,R2,R3]" : Inport  PortDimensions=3
  Fcn11 : Fcn  Expr=u(5)*u(4)
  Fcn12 : Fcn  Expr=u(5)*u(1)
  Fcn13 : Fcn  Expr=-u(2)
  Fcn21 : Fcn  Expr=u(3)*u(2)*u(4) - u(6)*u(1)
  Fcn22 : Fcn  Expr=u(3)*u(2)*u(1) + u(6)*u(4)
  Fcn23 : Fcn  Expr=u(3)*u(5)
  Fcn31 : Fcn  Expr=u(6)*u(2)*u(4) + u(3)*u(1)
  Fcn32 : Fcn  Expr=u(6)*u(2)*u(1) - u(3)*u(4)
  Fcn33 : Fcn  Expr=u(6)*u(5)
  Mux : Mux  Inputs=2
  Subsystem : Subsystem
  sincos : Trigonometry  Operator=sincos
  DCMbe : Outport  PortDimensions=[3,3]
  wires:
  sincos/1 -> Mux/1
  Subsystem/1(Matrix) -> DCMbe/1
  Fcn33/1 -> Subsystem/9(M33)
  Fcn13/1 -> Subsystem/3(M13)
  Fcn31/1 -> Subsystem/7(M31)
  Fcn32/1 -> Subsystem/8(M32)
  Fcn22/1 -> Subsystem/5(M22)
  Fcn12/1 -> Subsystem/2(M12)
  Fcn23/1 -> Subsystem/6(M23)
  Fcn21/1 -> Subsystem/4(M21)
  sincos/2 -> Mux/2
  Mux/1 -> Fcn22/1, Fcn23/1, Fcn31/1, Fcn33/1, Fcn32/1, Fcn21/1, Fcn13/1, Fcn12/1, Fcn11/1
  Fcn11/1 -> Subsystem/1(M11)
  "[R1,R2,R3]"/1 -> sincos/1

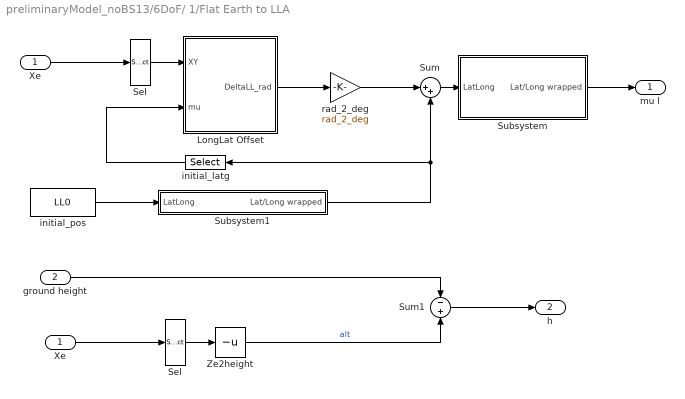
== system preliminaryModel_noBS13/6DoF/ 1/Flat Earth to LLA ==
  Xe : Inport
  ground height : Inport  Port=2
  LongLat Offset : Subsystem
  Sel : Selector  InputPortWidth=3  IndexOptions=Index vector (dialog)  Indices=[1,2]  OutputSizes=1
  "Sel " : Selector  InputPortWidth=3  IndexOptions=Index vector (dialog)  Indices=3  OutputSizes=1
  Subsystem : Subsystem
  Subsystem1 : Subsystem
  Sum : Sum  Inputs=|++
  Sum1 : Sum  Inputs=-+
  "Xe " : InportShadow
  Ze2height : UnaryMinus
  initial_latg : Selector  InputPortWidth=2  IndexOptions=Index vector (dialog)  Indices=[1]  OutputSizes=1
  initial_pos : Constant  Value=LL0
  rad_2_deg : Gain  Gain=rad_2_deg
  mu l : Outport
  h : Outport  Port=2
  wires:
  initial_pos/1 -> Subsystem1/1(LatLong)
  Sum/1 -> Subsystem/1(LatLong)
  ground height/1 -> Sum1/1
  Sel/1 -> LongLat Offset/1(XY)
  "Sel "/1 -> Ze2height/1
  Xe/1 -> Sel/1
  rad_2_deg/1 -> Sum/1
  "Xe "/1 -> "Sel "/1
  Subsystem1/1(Lat/Long wrapped) -> initial_latg/1, Sum/2
  initial_latg/1 -> LongLat Offset/2(mu)
  Ze2height/1 -> Sum1/2  "alt"
  Sum1/1 -> h/1
  Subsystem/1(Lat/Long wrapped) -> mu l/1
  LongLat Offset/1(DeltaLL_rad) -> rad_2_deg/1

== system preliminaryModel_noBS13/6DoF/6DOF/Calculate omega_dot ==
  p q r : Inport
  "I, I_dot" : Inport  Port=2
  Moments : Inport  Port=3
  I x w : Subsystem
  I x w1 : Subsystem
  Product2 : Product  Inputs=*/  Multiplication=Matrix(*)  SaturateOnIntegerOverflow=on  OutDataTypeStr=Inherit: Same as first input
  Reshape : Reshape
  Reshape1 : Reshape  OutputDimensionality=Row vector (2-D)
  Selector : Selector  NumberOfDimensions=2  InputPortWidth=2  IndexOptions=Index vector (dialog),Select all  Indices=1:3,-1  OutputSizes=1
  Selector1 : Selector  NumberOfDimensions=2  InputPortWidth=2  IndexOptions=Index vector (dialog),Select all  Indices=4:6,-1  OutputSizes=1
  Selector2 : Selector  NumberOfDimensions=2  InputPortWidth=2  IndexOptions=Index vector (dialog),Select all  Indices=1:3,-1  OutputSizes=1
  Sum2 : Sum  Inputs=+--  SaturateOnIntegerOverflow=on
  wx(Iw) : Subsystem
  pdot qdot rdot : Outport
  wires:
  Reshape1/1 -> Product2/1
  I x w/1(I * w) -> wx(Iw)/2(B)
  wx(Iw)/1(C) -> Sum2/3
  Selector1/1 -> I x w1/1(I_dot)
  I x w1/1(Id * w) -> Sum2/2
  Moments/1 -> Sum2/1
  Sum2/1 -> Reshape1/1
  Product2/1 -> Reshape/1
  p q r/1 -> I x w1/2(p q r), wx(Iw)/1(A), I x w/1(p q r)
  "I, I_dot"/1 -> Selector2/1, Selector/1, Selector1/1
  Selector2/1 -> Product2/2
  Selector/1 -> I x w/2(Inertia)
  Reshape/1 -> pdot qdot rdot/1

== system preliminaryModel_noBS13/6DoF/6DOF/Mass & Inertia ==
  Constant : Constant  Value=eye(3)  OutDataTypeStr=double
  Constant2 : Constant  Value=zeros(3)  OutDataTypeStr=double
  Vector Concatenate : Concatenate  Mode=Multidimensional array
  mass1 : Integrator  InitialCondition=mass  LimitOutput=on  UpperSaturationLimit=mass_f  LowerSaturationLimit=mass_e
  massflow : Constant  Value=m_dot  OutDataTypeStr=Inherit: Inherit via back propagation
  Mass : Outport
  Inertia : Outport  Port=2
  wires:
  Constant2/1 -> Vector Concatenate/2
  Constant/1 -> Vector Concatenate/1
  massflow/1 -> mass1/1
  Vector Concatenate/1 -> Inertia/1
  mass1/1 -> Mass/1

== system preliminaryModel_noBS13/6DoF/6DOF/Subsystem ==
  note: Rotation order ZYX
  "p q r " : Inport
  Rotation Angles to Direction Cosine Matrix : Subsystem
  Selector : Selector  InputPortWidth=3  IndexOptions=Index vector (dialog)  Indices=[3 2 1]  OutputSizes=1
  Subsystem : Subsystem
  phi theta psi : Integrator  InitialCondition=eul_0
  DCM : Outport
  Euler : Outport  Port=2
  wires:
  Selector/1 -> Rotation Angles to Direction Cosine Matrix/1("[R1,R2,R3]")
  "p q r "/1 -> Subsystem/1(p q r)
  phi theta psi/1 -> Subsystem/2(phi theta psi1), Euler/1, Selector/1
  Subsystem/1(phidot thetadot psi) -> phi theta psi/1
  Rotation Angles to Direction Cosine Matrix/1(DCMbe) -> DCM/1

== system preliminaryModel_noBS13/6DoF/6DOF/Subsystem1 ==
  x y z : Inport
  transform coefficients : Inport  Port=2
  Product1 : Product  Multiplication=Matrix(*)  SaturateOnIntegerOverflow=on  InputSameDT=on  OutDataTypeStr=Inherit: Same as first input
  Reshape1 : Reshape  OutputDimensionality=Column vector (2-D)
  Reshape2 : Reshape
  Ve : Outport
  wires:
  Reshape2/1 -> Ve/1
  transform coefficients/1 -> Product1/1
  x y z/1 -> Reshape1/1
  Reshape1/1 -> Product1/2
  Product1/1 -> Reshape2/1

== system preliminaryModel_noBS13/6DoF/6DOF/Vbxw ==
  A : Inport
  B : Inport  Port=2
  "A " : InportShadow
  "B " : InportShadow  Port=2
  Subsystem : Subsystem
  Subsystem1 : Subsystem
  Sum : Sum  Inputs=+|-  SaturateOnIntegerOverflow=on  InputSameDT=on  OutDataTypeStr=Inherit: Same as first input
  C : Outport
  wires:
  "B "/1 -> Subsystem1/2(B)
  "A "/1 -> Subsystem1/1(A)
  Sum/1 -> C/1
  B/1 -> Subsystem/2(B)
  A/1 -> Subsystem/1(A)
  Subsystem/1(Out1) -> Sum/1
  Subsystem1/1(Out1) -> Sum/2

== system preliminaryModel_noBS13/Aerodynamics/Control stab/Subsystem ==
  note: delta angle in
  Canard Actions : Inport
  Elevon 1 : Inport  Port=2
  Elevon 2 : Inport  Port=3
  Rudder : Inport  Port=4
  Canard : Subsystem
  Control deriv tot : Sum  Inputs=++++  SaturateOnIntegerOverflow=on  InputSameDT=on  OutDataTypeStr=Inherit: Same as first input
  "Elevon 1 " : Subsystem
  "Elevon 2 " : Subsystem
  "Rudder " : Subsystem
  Control Derivatives : Outport
  wires:
  Elevon 1/1 -> "Elevon 1 "/1(In1)
  Elevon 2/1 -> "Elevon 2 "/1(In1)
  Canard Actions/1 -> Canard/1(In1)
  Rudder/1 -> "Rudder "/1(In1)
  Canard/1(DerivCanard) -> Control deriv tot/1
  "Elevon 1 "/1(DerivElevonPort) -> Control deriv tot/2
  "Elevon 2 "/1(DerivElevonStar) -> Control deriv tot/3
  "Rudder "/1(DerivRudder) -> Control deriv tot/4
  Control deriv tot/1 -> Control Derivatives/1

== system preliminaryModel_noBS13/Aerodynamics/Subsystem5/3x3 Cross Product ==
  A : Inport
  B : Inport  Port=2
  A_1 : InportShadow
  B_1 : InportShadow  Port=2
  Subsystem1 : Subsystem
  Subsystem3 : Subsystem
  Sum : Sum  Inputs=+|-  SaturateOnIntegerOverflow=on  InputSameDT=on  OutDataTypeStr=Inherit: Same as first input
  C : Outport
  wires:
  Sum/1 -> C/1
  B/1 -> Subsystem1/2(B)
  Subsystem3/1(Out1) -> Sum/2
  A/1 -> Subsystem1/1(A)
  Subsystem1/1(Out1) -> Sum/1
  B_1/1 -> Subsystem3/2(B)
  A_1/1 -> Subsystem3/1(A)

== system preliminaryModel_noBS13/Aerodynamics/Subsystem5/Subsystem ==
  Vb1 : Inport
  In_w : Inport  Port=2
  Mux : Mux  Inputs=2
  Product : Product  Multiplication=Matrix(*)  RndMeth=Zero
  Subsystem : Subsystem
  Subsystem1 : Subsystem
  Terminator1 : Terminator
  Transpose : Math  Operator=transpose  SaturateOnIntegerOverflow=on
  Out_b : Outport
  wires:
  Product/1 -> Out_b/1
  Subsystem/1(DCM) -> Transpose/1
  Subsystem1/3(V) -> Terminator1/1
  Mux/1 -> Subsystem/1(alpha beta)
  Vb1/1 -> Subsystem1/1(Vb)
  Subsystem1/1(Alpha) -> Mux/1
  Subsystem1/2(Beta) -> Mux/2
  In_w/1 -> Product/2
  Transpose/1 -> Product/1

== system preliminaryModel_noBS13/Aerodynamics/Subsystem5/Subsystem2 ==
  Vb1 : Inport
  In_w : Inport  Port=2
  Mux : Mux  Inputs=2
  Product : Product  Multiplication=Matrix(*)  RndMeth=Zero
  Subsystem : Subsystem
  Subsystem1 : Subsystem
  Terminator1 : Terminator
  Transpose : Math  Operator=transpose  SaturateOnIntegerOverflow=on
  Out_b : Outport
  wires:
  Product/1 -> Out_b/1
  Subsystem/1(DCM) -> Transpose/1
  Subsystem1/3(V) -> Terminator1/1
  Mux/1 -> Subsystem/1(alpha beta)
  Vb1/1 -> Subsystem1/1(Vb)
  Subsystem1/1(Alpha) -> Mux/1
  Subsystem1/2(Beta) -> Mux/2
  In_w/1 -> Product/2
  Transpose/1 -> Product/1

== system preliminaryModel_noBS13/Aerodynamics/Subsystem5/Subsystem3 ==
  Vb1 : Inport
  In_w : Inport  Port=2
  Mux : Mux  Inputs=2
  Product : Product  Multiplication=Matrix(*)  RndMeth=Zero
  Subsystem : Subsystem
  Subsystem1 : Subsystem
  Terminator1 : Terminator
  Transpose : Math  Operator=transpose  SaturateOnIntegerOverflow=on
  Out_b : Outport
  wires:
  Product/1 -> Out_b/1
  Subsystem/1(DCM) -> Transpose/1
  Subsystem1/3(V) -> Terminator1/1
  Mux/1 -> Subsystem/1(alpha beta)
  Vb1/1 -> Subsystem1/1(Vb)
  Subsystem1/1(Alpha) -> Mux/1
  Subsystem1/2(Beta) -> Mux/2
  In_w/1 -> Product/2
  Transpose/1 -> Product/1

== system preliminaryModel_noBS13/3DOF/Transform to Earth Axes/Rotation Angles to Direction Cosine Matrix/Subsystem ==
  M11 : Inport  PortDimensions=1
  M12 : Inport  Port=2  PortDimensions=1
  M13 : Inport  Port=3  PortDimensions=1
  M21 : Inport  Port=4  PortDimensions=1
  M22 : Inport  Port=5  PortDimensions=1
  M23 : Inport  Port=6  PortDimensions=1
  M31 : Inport  Port=7  PortDimensions=1
  M32 : Inport  Port=8  PortDimensions=1
  M33 : Inport  Port=9  PortDimensions=1
  Reshape (9) to [3x3] column-major : Reshape  OutputDimensionality=Customize  OutputDimensions=[3,3]
  Vector Concatenate : Concatenate  NumInputs=9
  Matrix : Outport  PortDimensions=[3 3]
  wires:
  M23/1 -> Vector Concatenate/8
  M13/1 -> Vector Concatenate/7
  M32/1 -> Vector Concatenate/6
  Reshape (9) to [3x3] column-major/1 -> Matrix/1
  M22/1 -> Vector Concatenate/5
  M12/1 -> Vector Concatenate/4
  M31/1 -> Vector Concatenate/3
  M11/1 -> Vector Concatenate/1
  Vector Concatenate/1 -> Reshape (9) to [3x3] column-major/1
  M21/1 -> Vector Concatenate/2
  M33/1 -> Vector Concatenate/9

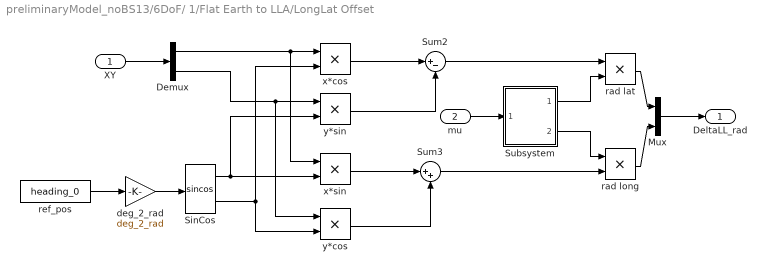
== system preliminaryModel_noBS13/6DoF/ 1/Flat Earth to LLA/LongLat Offset ==
  XY : Inport
  mu : Inport  Port=2
  Demux : Demux  Outputs=2
  Mux : Mux  Inputs=2
  SinCos : Trigonometry  Operator=sincos
  Subsystem : Subsystem
  Sum2 : Sum  Inputs=|+-
  Sum3 : Sum  Inputs=|++
  deg_2_rad : Gain  Gain=deg_2_rad
  rad lat : Product  RndMeth=Zero
  "rad long " : Product  RndMeth=Zero
  ref_pos : Constant  Value=heading_0
  x*cos : Product  RndMeth=Zero
  x*sin : Product  RndMeth=Zero
  y*cos : Product  RndMeth=Zero
  y*sin : Product  RndMeth=Zero
  DeltaLL_rad : Outport
  wires:
  mu/1 -> Subsystem/1(mu1)
  Subsystem/1(dNorth) -> rad lat/2
  Subsystem/2(dEast) -> "rad long "/1
  rad lat/1 -> Mux/1
  "rad long "/1 -> Mux/2
  Mux/1 -> DeltaLL_rad/1
  deg_2_rad/1 -> SinCos/1
  Demux/2 -> y*cos/1, y*sin/1
  Sum3/1 -> "rad long "/2
  y*cos/1 -> Sum3/2
  x*sin/1 -> Sum3/1
  Sum2/1 -> rad lat/1
  y*sin/1 -> Sum2/2
  SinCos/1 -> x*sin/2, y*sin/2
  x*cos/1 -> Sum2/1
  SinCos/2 -> y*cos/2, x*cos/2
  Demux/1 -> x*sin/1, x*cos/1
  XY/1 -> Demux/1
  ref_pos/1 -> deg_2_rad/1

== system preliminaryModel_noBS13/6DoF/ 1/Flat Earth to LLA/Subsystem ==
  LatLong : Inport
  Constant : Constant  Value=180
  Constant1 : Constant  Value=0
  Demux : Demux  Outputs=2
  Latitude Wrap 90 : Subsystem
  Mux : Mux  Inputs=2
  Sum2 : Sum  Inputs=|++
  Switch1 : Switch  Criteria=u2 ~= 0
  Wrap Longitude : Subsystem
  Lat/Long wrapped : Outport
  wires:
  Mux/1 -> Lat/Long wrapped/1
  Latitude Wrap 90/1(Lat wrapped) -> Mux/1
  Latitude Wrap 90/2(Wrap flag) -> Switch1/2
  Demux/1 -> Latitude Wrap 90/1(Lat)
  Demux/2 -> Sum2/2
  Sum2/1 -> Wrap Longitude/1(Angle)
  Wrap Longitude/1(Angle 180) -> Mux/2
  Constant/1 -> Switch1/1
  LatLong/1 -> Demux/1
  Constant1/1 -> Switch1/3
  Switch1/1 -> Sum2/1

== system preliminaryModel_noBS13/6DoF/ 1/Flat Earth to LLA/Subsystem1 ==
  LatLong : Inport
  Constant : Constant  Value=180
  Constant1 : Constant  Value=0
  Demux : Demux  Outputs=2
  Latitude Wrap 90 : Subsystem
  Mux : Mux  Inputs=2
  Sum2 : Sum  Inputs=|++
  Switch1 : Switch  Criteria=u2 ~= 0
  Wrap Longitude : Subsystem
  Lat/Long wrapped : Outport
  wires:
  Wrap Longitude/1(Angle 180) -> Mux/2
  LatLong/1 -> Demux/1
  Latitude Wrap 90/1(Lat wrapped) -> Mux/1
  Constant/1 -> Switch1/1
  Constant1/1 -> Switch1/3
  Demux/1 -> Latitude Wrap 90/1(Lat)
  Mux/1 -> Lat/Long wrapped/1
  Latitude Wrap 90/2(Wrap flag) -> Switch1/2
  Demux/2 -> Sum2/2
  Switch1/1 -> Sum2/1
  Sum2/1 -> Wrap Longitude/1(Angle)

== system preliminaryModel_noBS13/6DoF/6DOF/Calculate omega_dot/I x w ==
  p q r : Inport
  Inertia : Inport  Port=2
  Product : Product  Multiplication=Matrix(*)  SaturateOnIntegerOverflow=on  InputSameDT=on  OutDataTypeStr=Inherit: Same as first input
  Reshape1 : Reshape  OutputDimensionality=Column vector (2-D)
  Reshape2 : Reshape
  I * w : Outport
  wires:
  Reshape2/1 -> I * w/1
  Reshape1/1 -> Product/2
  p q r/1 -> Reshape1/1
  Inertia/1 -> Product/1
  Product/1 -> Reshape2/1

== system preliminaryModel_noBS13/6DoF/6DOF/Calculate omega_dot/I x w1 ==
  I_dot : Inport
  p q r : Inport  Port=2
  Product : Product  Multiplication=Matrix(*)  SaturateOnIntegerOverflow=on  InputSameDT=on  OutDataTypeStr=Inherit: Same as first input
  Reshape1 : Reshape  OutputDimensionality=Column vector (2-D)
  Reshape2 : Reshape
  Id * w : Outport
  wires:
  Reshape2/1 -> Id * w/1
  Reshape1/1 -> Product/2
  Product/1 -> Reshape2/1
  I_dot/1 -> Product/1
  p q r/1 -> Reshape1/1

== system preliminaryModel_noBS13/6DoF/6DOF/Calculate omega_dot/wx(Iw) ==
  A : Inport
  B : Inport  Port=2
  "A " : InportShadow
  "B " : InportShadow  Port=2
  Subsystem : Subsystem
  Subsystem1 : Subsystem
  Sum : Sum  Inputs=+|-  SaturateOnIntegerOverflow=on  InputSameDT=on  OutDataTypeStr=Inherit: Same as first input
  C : Outport
  wires:
  "B "/1 -> Subsystem1/2(B)
  "A "/1 -> Subsystem1/1(A)
  Sum/1 -> C/1
  B/1 -> Subsystem/2(B)
  A/1 -> Subsystem/1(A)
  Subsystem/1(Out1) -> Sum/1
  Subsystem1/1(Out1) -> Sum/2

== system preliminaryModel_noBS13/6DoF/6DOF/Subsystem/Rotation Angles to Direction Cosine Matrix ==
  "[R1,R2,R3]" : Inport  PortDimensions=3
  Fcn11 : Fcn  Expr=u(5)*u(4)
  Fcn12 : Fcn  Expr=u(5)*u(1)
  Fcn13 : Fcn  Expr=-u(2)
  Fcn21 : Fcn  Expr=u(3)*u(2)*u(4) - u(6)*u(1)
  Fcn22 : Fcn  Expr=u(3)*u(2)*u(1) + u(6)*u(4)
  Fcn23 : Fcn  Expr=u(3)*u(5)
  Fcn31 : Fcn  Expr=u(6)*u(2)*u(4) + u(3)*u(1)
  Fcn32 : Fcn  Expr=u(6)*u(2)*u(1) - u(3)*u(4)
  Fcn33 : Fcn  Expr=u(6)*u(5)
  Mux : Mux  Inputs=2
  Subsystem : Subsystem
  sincos : Trigonometry  Operator=sincos
  DCMbe : Outport  PortDimensions=[3,3]
  wires:
  "[R1,R2,R3]"/1 -> sincos/1
  Fcn11/1 -> Subsystem/1(M11)
  Mux/1 -> Fcn11/1, Fcn12/1, Fcn13/1, Fcn21/1, Fcn32/1, Fcn33/1, Fcn31/1, Fcn23/1, Fcn22/1
  sincos/2 -> Mux/2
  Fcn21/1 -> Subsystem/4(M21)
  Fcn23/1 -> Subsystem/6(M23)
  Fcn12/1 -> Subsystem/2(M12)
  Fcn22/1 -> Subsystem/5(M22)
  Fcn32/1 -> Subsystem/8(M32)
  Fcn31/1 -> Subsystem/7(M31)
  Fcn13/1 -> Subsystem/3(M13)
  Fcn33/1 -> Subsystem/9(M33)
  Subsystem/1(Matrix) -> DCMbe/1
  sincos/1 -> Mux/1

== system preliminaryModel_noBS13/6DoF/6DOF/Subsystem/Subsystem ==
  p q r : Inport
  phi theta psi1 : Inport  Port=2
  Mux1 : Mux  Inputs=[3 3 3]
  Mux2 : Mux  Inputs=3
  phidot : Fcn  Expr=u[1]+(u[2]*u[4]+u[3]*u[7])*(u[5]/u[8])
  psidot : Fcn  Expr=(u[2]*u[4]+u[3]*u[7])/u[8]
  sincos : Trigonometry  Operator=sincos
  thetadot : Fcn  Expr=u[2]*u[7]-u[3]*u[4]
  phidot thetadot psi : Outport  InitialOutput=0
  wires:
  sincos/1 -> Mux1/2
  psidot/1 -> Mux2/3
  Mux2/1 -> phidot thetadot psi/1
  phidot/1 -> Mux2/1
  sincos/2 -> Mux1/3
  thetadot/1 -> Mux2/2
  phi theta psi1/1 -> sincos/1
  p q r/1 -> Mux1/1
  Mux1/1 -> psidot/1, phidot/1, thetadot/1

== system preliminaryModel_noBS13/6DoF/6DOF/Vbxw/Subsystem ==
  A : Inport
  B : Inport  Port=2
  Demux : Demux  Outputs=3
  Demux1 : Demux  Outputs=3
  Mux : Mux  Inputs=3
  i x j : Product  SaturateOnIntegerOverflow=on  InputSameDT=on  OutDataTypeStr=Inherit: Same as first input
  j x k : Product  SaturateOnIntegerOverflow=on  InputSameDT=on  OutDataTypeStr=Inherit: Same as first input
  k x i : Product  SaturateOnIntegerOverflow=on  InputSameDT=on  OutDataTypeStr=Inherit: Same as first input
  Out1 : Outport
  wires:
  Demux1/3 -> j x k/2
  Demux/2 -> j x k/1
  Demux/3 -> k x i/1
  Demux1/1 -> k x i/2
  Demux1/2 -> i x j/2
  Demux/1 -> i x j/1
  i x j/1 -> Mux/3
  k x i/1 -> Mux/2
  j x k/1 -> Mux/1
  B/1 -> Demux1/1
  A/1 -> Demux/1
  Mux/1 -> Out1/1

== system preliminaryModel_noBS13/6DoF/6DOF/Vbxw/Subsystem1 ==
  A : Inport
  B : Inport  Port=2
  Demux : Demux  Outputs=3
  Demux1 : Demux  Outputs=3
  Mux : Mux  Inputs=3
  i x k : Product  SaturateOnIntegerOverflow=on  InputSameDT=on  OutDataTypeStr=Inherit: Same as first input
  j x i : Product  SaturateOnIntegerOverflow=on  InputSameDT=on  OutDataTypeStr=Inherit: Same as first input
  k x j : Product  SaturateOnIntegerOverflow=on  InputSameDT=on  OutDataTypeStr=Inherit: Same as first input
  Out1 : Outport
  wires:
  j x i/1 -> Mux/3
  i x k/1 -> Mux/2
  k x j/1 -> Mux/1
  Mux/1 -> Out1/1
  Demux1/1 -> j x i/2
  Demux/2 -> j x i/1
  Demux1/3 -> i x k/2
  Demux/1 -> i x k/1
  Demux1/2 -> k x j/2
  Demux/3 -> k x j/1
  B/1 -> Demux1/1
  A/1 -> Demux/1
